simulink model "Task2_2"  (R2021a)
settings: Solver=VariableStepAuto  StartTime=0.0  StopTime=stop_time  RelTol=1e-3
values from neighbouring files (symbols this model uses):
  i_sd_ref = i_sd_mat(end)    [Code2021_Jo_Saleh.m]    (also in ExeRet21.m.m)
  i_sq_ref = i_sq_mat(end)    [Code2021_Jo_Saleh.m]    (also in ExeRet21.m.m)
  Kd_i = Rs * Kd_p / Lsd    (= -20)    [Code2021_Jo_Saleh.m]    (also in ExeRet21.m.m)
  Kd_p = - Lsd / tau_i    (= -2)    [Code2021_Jo_Saleh.m]    (also in ExeRet21.m.m)
  Kq_i = Rs * Kq_p / Lsq    (= -20)    [Code2021_Jo_Saleh.m]    (also in ExeRet21.m.m)
  Kq_p = - Lsq / tau_i    (= -2.66666666667)    [Code2021_Jo_Saleh.m]    (also in ExeRet21.m.m)
  Lsd = 6e-3    (= 0.006)    [Code2021_Jo_Saleh.m]    (also in ExeRet21.m.m)
  Lsq = 8e-3    (= 0.008)    [Code2021_Jo_Saleh.m]    (also in ExeRet21.m.m)
  Phi_m = 17.3    [Code2021_Jo_Saleh.m]    (also in ExeRet21.m.m)
  Ptur = 3.5e6    (= 3500000)    [Code2021_Jo_Saleh.m]    (also in ExeRet21.m.m)
  Rs = 60e-3    (= 0.06)    [Code2021_Jo_Saleh.m]    (also in ExeRet21.m.m)
  Vdc = 6e3    (= 6000)    [Code2021_Jo_Saleh.m]    (also in ExeRet21.m.m)
  we = wm * (p / 2)    (= 188.495559215)    [Code2021_Jo_Saleh.m]    (also in ExeRet21.m.m)
libraries: pid_lib x2
settings Model: Creator=Tomo  LastModifiedBy=Tomo
settings SolverCC: AlgebraicLoopSolver=TrustRegion
settings DebuggingCC: SFMachineParentedDataDiag=warning

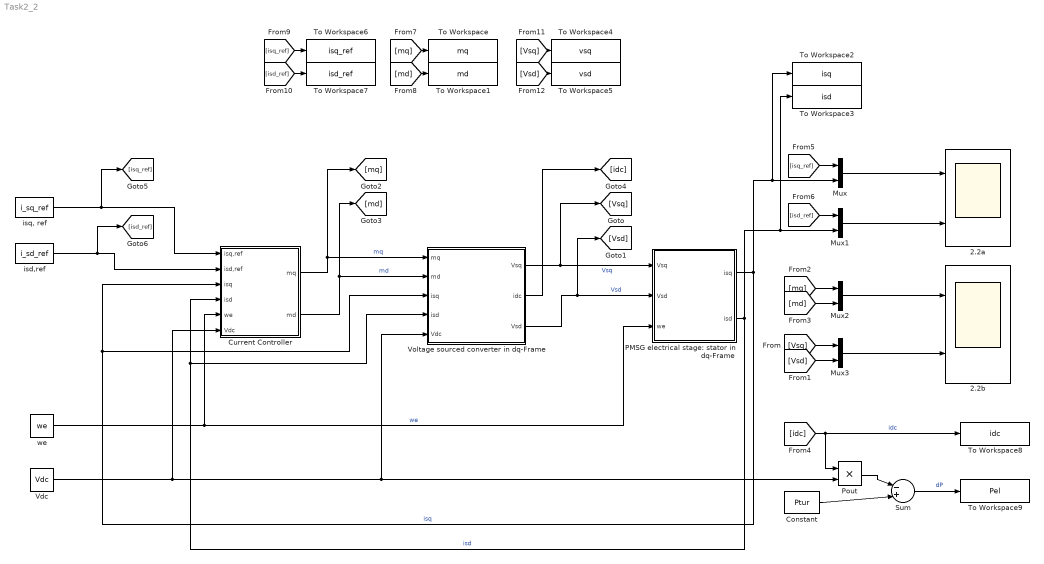
== system Task2_2 ==
  2.2a : Scope  NumInputPorts=2
  2.2b : Scope  NumInputPorts=2
  Constant : Constant  Value=Ptur
  Current Controller : Subsystem
  Mux{,1..3} (4 alike) : Mux  Inputs=2
  PMSG electrical stage: stator in dq-Frame : Subsystem
  Pout : Product
  Sum : Sum  Inputs=|-+|
  To Workspace : ToWorkspace  VariableName=mq  SampleTime=-1
  To Workspace1 : ToWorkspace  VariableName=md  SampleTime=-1
  To Workspace2 : ToWorkspace  VariableName=isq  SampleTime=-1
  To Workspace3 : ToWorkspace  VariableName=isd  SampleTime=-1
  To Workspace4 : ToWorkspace  VariableName=vsq  SampleTime=-1
  To Workspace5 : ToWorkspace  VariableName=vsd  SampleTime=-1
  To Workspace6 : ToWorkspace  VariableName=isq_ref  SampleTime=-1
  To Workspace7 : ToWorkspace  VariableName=isd_ref  SampleTime=-1
  To Workspace8 : ToWorkspace  VariableName=idc  SampleTime=-1
  To Workspace9 : ToWorkspace  VariableName=Pel  SampleTime=-1
  Vdc : Constant  Value=Vdc
  Voltage sourced converter in dq-Frame : Subsystem
  isd,ref : Constant  Value=i_sd_ref
  "isq, ref" : Constant  Value=i_sq_ref
  we : Constant  Value=we
  wires:
  "isq, ref"/1 -> [isq_ref], Current Controller/1(isq,ref)
  isd,ref/1 -> [isd_ref], Current Controller/2(isd,ref)
  PMSG electrical stage: stator in dq-Frame/1(isq) -> To Workspace2/1, Mux/2, Voltage sourced converter in dq-Frame/3(isq), Current Controller/3(isq)  "isq"
  PMSG electrical stage: stator in dq-Frame/2(isd) -> To Workspace3/1, Mux1/2, Voltage sourced converter in dq-Frame/4(isd), Current Controller/4(isd)  "isd"
  we/1 -> PMSG electrical stage: stator in dq-Frame/3(we), Current Controller/5(we)  "we"
  Vdc/1 -> Voltage sourced converter in dq-Frame/5(Vdc), Pout/2, Current Controller/6(Vdc)
  Current Controller/1(mq) -> [mq], Voltage sourced converter in dq-Frame/1(mq)  "mq"
  Current Controller/2(md) -> [md], Voltage sourced converter in dq-Frame/2(md)  "md"
  Voltage sourced converter in dq-Frame/1(Vsq) -> PMSG electrical stage: stator in dq-Frame/1(Vsq), [Vsq]  "Vsq"
  Voltage sourced converter in dq-Frame/3(Vsd) -> [Vsd], PMSG electrical stage: stator in dq-Frame/2(Vsd)  "Vsd"
  [Vsq] -> Mux3/1
  Voltage sourced converter in dq-Frame/2(idc) -> [idc]
  [idc] -> To Workspace8/1, Pout/1  "idc"
  [isq_ref] -> Mux/1
  Mux/1 -> 2.2a/1
  Mux1/1 -> 2.2a/2
  [isd_ref] -> Mux1/1
  Mux2/1 -> 2.2b/1
  Mux3/1 -> 2.2b/2
  [Vsd] -> Mux3/2
  [md] -> Mux2/2
  [mq] -> Mux2/1
  Constant/1 -> Sum/2
  Pout/1 -> Sum/1
  Sum/1 -> To Workspace9/1  "dP"
  [mq] -> To Workspace/1
  [md] -> To Workspace1/1
  [Vsd] -> To Workspace5/1
  [Vsq] -> To Workspace4/1
  [isq_ref] -> To Workspace6/1
  [isd_ref] -> To Workspace7/1

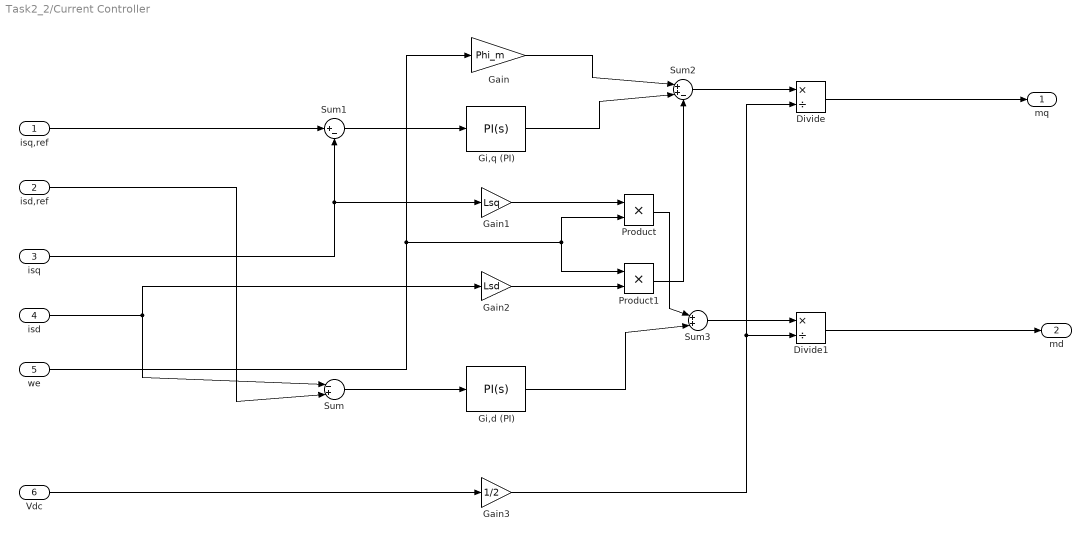
== system Task2_2/Current Controller ==
  isq,ref : Inport
  isd,ref : Inport  Port=2
  isq : Inport  Port=3
  isd : Inport  Port=4
  we : Inport  Port=5
  Vdc : Inport  Port=6
  Divide : Product  Inputs=*/
  Divide1 : Product  Inputs=*/
  Gain : Gain  Gain=Phi_m
  Gain1 : Gain  Gain=Lsq
  Gain2 : Gain  Gain=Lsd
  Gain3 : Gain  Gain=1/2
  Gi,d (PI) : pid_lib/PID Controller  Controller=PI  Form=Parallel  TimeDomain=Continuous-time  UseExternalTs=off  SampleTime=-1  IntegratorMethod=Forward Euler  FilterMethod=Forward Euler  ControllerParametersSource=internal  P=Kd_p  I=Kd_i  D=0  UseFilter=on  N=100  TunerSelectOption=Transfer Function Based (PID Tuner App)  InitialConditionSource=internal  InitialConditionForIntegrator=0  InitialConditionForFilter=0  DifferentiatorICPrevScaledInput=0  ExternalReset=none  TrackingMode=off  Kt=1  LimitOutput=off  SatLimitsSource=internal  UpperSaturationLimit=inf  LowerSaturationLimit=-inf  LinearizeAsGain=on  AntiWindupMode=none  Kb=1  POutMin=[]  POutMax=[]  IOutMin=[]  IOutMax=[]  DOutMin=[]  DOutMax=[]  NOutMin=[]  NOutMax=[]  SumOutMin=[]  SumOutMax=[]  SaturationOutMin=[]  SaturationOutMax=[]  PParamMin=[]  PParamMax=[]  IParamMin=[]  IParamMax=[]  DParamMin=[]  DParamMax=[]  NParamMin=[]  NParamMax=[]  KbParamMin=[]  KbParamMax=[]  KtParamMin=[]  KtParamMax=[]  KbOutMin=[]  KbOutMax=[]  KtOutMin=[]  KtOutMax=[]  IntegratorOutMin=[]  IntegratorOutMax=[]  FilterOutMin=[]  FilterOutMax=[]  SumI1OutMin=[]  SumI1OutMax=[]  SumI2OutMin=[]  SumI2OutMax=[]  SumI3OutMin=[]  SumI3OutMax=[]  SumI4OutMin=[]  SumI4OutMax=[]  SumDOutMin=[]  SumDOutMax=[]  DifferentiatorOutMin=[]  DifferentiatorOutMax=[]  FilterDiffOutCoefMin=[]  FilterDiffOutCoefMax=[]  ReciprocalOutMin=[]  ReciprocalOutMax=[]  SumDenOutMin=[]  SumDenOutMax=[]  SumNumOutMin=[]  SumNumOutMax=[]  DivideOutMin=[]  DivideOutMax=[]  UdiffTsProdOutMin=[]  UdiffTsProdOutMax=[]  NTsProdOutMin=[]  NTsProdOutMax=[]  UintegralTsProdOutMin=[]  UintegralTsProdOutMax=[]  UngainTsProdOutMin=[]  UngainTsProdOutMax=[]  IntegratorContinuousStateAttributes=''  IntegratorStateMustResolveToSignalObject=off  IntegratorRTWStateStorageClass=Auto  FilterContinuousStateAttributes=''  FilterStateMustResolveToSignalObject=off  FilterRTWStateStorageClass=Auto  ParallelPVariant=InternalParameters  IdealPVariant=Disabled  IVariant=InternalParameters  DVariant=Disabled  IntegratorVariant=Continuous  SatVariant=Disabled  AWVariant=Passthrough  PCopyVariant=Disabled  TRVariant=Disabled  FdbkBlocksVariant=Forward  IdealPFdbkVariant=Disabled  SatFdbkVariant=Disabled  DerivativeFilterVariant=Disabled  NVariant=Disabled  NCopyVariant=Disabled_SignalSpec  FilterICVariant=Disabled  IntegratorICVariant=InternalICs  ExternalResetVariant=Disabled  TRSumVariant=Passthrough  SumFdbkVariant=Disabled  SumVariant=Sum_PI  TsampFilterVariant=InternalTs  TsampNgainVariant=Passthrough  TsampIntegralVariant=Passthrough  ExternalSaturationOutDataTypeStr=Inherit: Same as second input
  Gi,q (PI) : pid_lib/PID Controller  Controller=PI  Form=Parallel  TimeDomain=Continuous-time  UseExternalTs=off  SampleTime=-1  IntegratorMethod=Forward Euler  FilterMethod=Forward Euler  ControllerParametersSource=internal  P=Kq_p  I=Kq_i  D=0  UseFilter=on  N=100  TunerSelectOption=Transfer Function Based (PID Tuner App)  InitialConditionSource=internal  InitialConditionForIntegrator=0  InitialConditionForFilter=0  DifferentiatorICPrevScaledInput=0  ExternalReset=none  TrackingMode=off  Kt=1  LimitOutput=off  SatLimitsSource=internal  UpperSaturationLimit=inf  LowerSaturationLimit=-inf  LinearizeAsGain=on  AntiWindupMode=none  Kb=1  POutMin=[]  POutMax=[]  IOutMin=[]  IOutMax=[]  DOutMin=[]  DOutMax=[]  NOutMin=[]  NOutMax=[]  SumOutMin=[]  SumOutMax=[]  SaturationOutMin=[]  SaturationOutMax=[]  PParamMin=[]  PParamMax=[]  IParamMin=[]  IParamMax=[]  DParamMin=[]  DParamMax=[]  NParamMin=[]  NParamMax=[]  KbParamMin=[]  KbParamMax=[]  KtParamMin=[]  KtParamMax=[]  KbOutMin=[]  KbOutMax=[]  KtOutMin=[]  KtOutMax=[]  IntegratorOutMin=[]  IntegratorOutMax=[]  FilterOutMin=[]  FilterOutMax=[]  SumI1OutMin=[]  SumI1OutMax=[]  SumI2OutMin=[]  SumI2OutMax=[]  SumI3OutMin=[]  SumI3OutMax=[]  SumI4OutMin=[]  SumI4OutMax=[]  SumDOutMin=[]  SumDOutMax=[]  DifferentiatorOutMin=[]  DifferentiatorOutMax=[]  FilterDiffOutCoefMin=[]  FilterDiffOutCoefMax=[]  ReciprocalOutMin=[]  ReciprocalOutMax=[]  SumDenOutMin=[]  SumDenOutMax=[]  SumNumOutMin=[]  SumNumOutMax=[]  DivideOutMin=[]  DivideOutMax=[]  UdiffTsProdOutMin=[]  UdiffTsProdOutMax=[]  NTsProdOutMin=[]  NTsProdOutMax=[]  UintegralTsProdOutMin=[]  UintegralTsProdOutMax=[]  UngainTsProdOutMin=[]  UngainTsProdOutMax=[]  IntegratorContinuousStateAttributes=''  IntegratorStateMustResolveToSignalObject=off  IntegratorRTWStateStorageClass=Auto  FilterContinuousStateAttributes=''  FilterStateMustResolveToSignalObject=off  FilterRTWStateStorageClass=Auto  ParallelPVariant=InternalParameters  IdealPVariant=Disabled  IVariant=InternalParameters  DVariant=Disabled  IntegratorVariant=Continuous  SatVariant=Disabled  AWVariant=Passthrough  PCopyVariant=Disabled  TRVariant=Disabled  FdbkBlocksVariant=Forward  IdealPFdbkVariant=Disabled  SatFdbkVariant=Disabled  DerivativeFilterVariant=Disabled  NVariant=Disabled  NCopyVariant=Disabled_SignalSpec  FilterICVariant=Disabled  IntegratorICVariant=InternalICs  ExternalResetVariant=Disabled  TRSumVariant=Passthrough  SumFdbkVariant=Disabled  SumVariant=Sum_PI  TsampFilterVariant=InternalTs  TsampNgainVariant=Passthrough  TsampIntegralVariant=Passthrough  ExternalSaturationOutDataTypeStr=Inherit: Same as second input
  Product : Product
  Product1 : Product
  Sum : Sum  Inputs=|-+|
  Sum1 : Sum  Inputs=|+-
  Sum2 : Sum  Inputs=|++-
  Sum3 : Sum  Inputs=|++|
  mq : Outport
  md : Outport  Port=2
  wires:
  Gain3/1 -> Divide/2, Divide1/2
  we/1 -> Gain/1, Product1/1, Product/2
  Sum/1 -> Gi,d (PI)/1
  Vdc/1 -> Gain3/1
  Sum3/1 -> Divide1/1
  isq/1 -> Gain1/1, Sum1/2
  Sum1/1 -> Gi,q (PI)/1
  Gain/1 -> Sum2/1
  Gain2/1 -> Product1/2
  isd,ref/1 -> Sum/2
  Sum2/1 -> Divide/1
  Gi,d (PI)/1 -> Sum3/2
  Product/1 -> Sum3/1
  Product1/1 -> Sum2/3
  Gain1/1 -> Product/1
  isq,ref/1 -> Sum1/1
  Gi,q (PI)/1 -> Sum2/2
  Divide/1 -> mq/1
  isd/1 -> Gain2/1, Sum/1
  Divide1/1 -> md/1

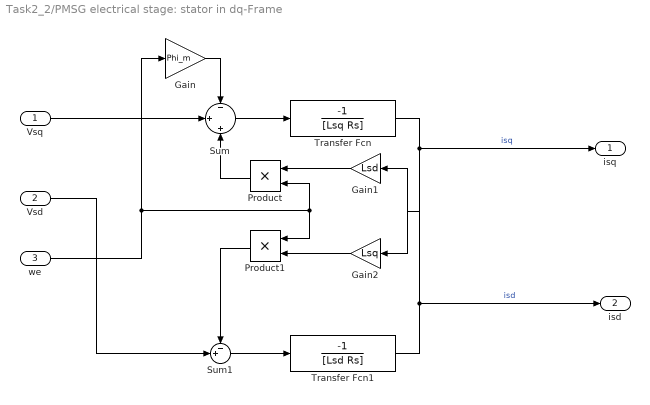
== system Task2_2/PMSG electrical stage: stator in dq-Frame ==
  Vsq : Inport
  Vsd : Inport  Port=2
  we : Inport  Port=3
  Gain : Gain  Gain=Phi_m
  Gain1 : Gain  Gain=Lsd
  Gain2 : Gain  Gain=Lsq
  Product : Product
  Product1 : Product
  Sum : Sum  Inputs=-|+|+
  Sum1 : Sum  Inputs=-+|
  Transfer Fcn : TransferFcn  Numerator=[-1]  Denominator=[Lsq Rs]
  Transfer Fcn1 : TransferFcn  Numerator=[-1]  Denominator=[Lsd Rs]
  isq : Outport
  isd : Outport  Port=2
  wires:
  Sum/1 -> Transfer Fcn/1
  Product/1 -> Sum/3
  Gain/1 -> Sum/1
  we/1 -> Gain/1, Product/2, Product1/1
  Transfer Fcn1/1 -> Gain1/1, isd/1  "isd"
  Vsq/1 -> Sum/2
  Transfer Fcn/1 -> Gain2/1, isq/1  "isq"
  Product1/1 -> Sum1/1
  Sum1/1 -> Transfer Fcn1/1
  Vsd/1 -> Sum1/2
  Gain1/1 -> Product/1
  Gain2/1 -> Product1/2

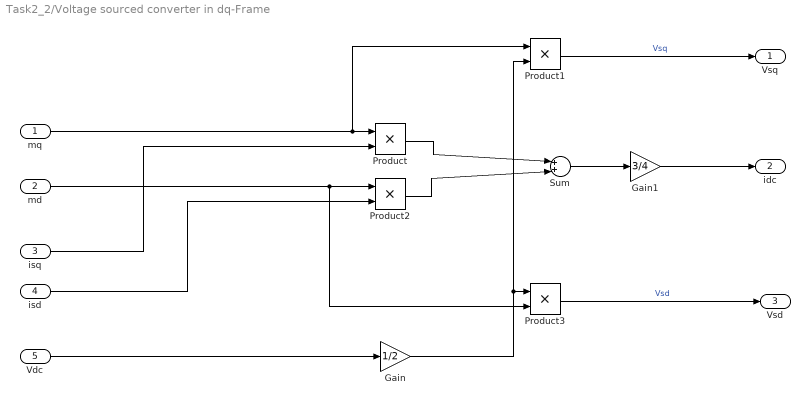
== system Task2_2/Voltage sourced converter in dq-Frame ==
  mq : Inport
  md : Inport  Port=2
  isq : Inport  Port=3
  isd : Inport  Port=4
  Vdc : Inport  Port=5
  Gain : Gain  Gain=1/2
  Gain1 : Gain  Gain=3/4
  Product{,1..3} (4 alike) : Product
  Sum : Sum  Inputs=|++|
  Vsq : Outport
  idc : Outport  Port=2
  Vsd : Outport  Port=3
  wires:
  Product2/1 -> Sum/2
  mq/1 -> Product1/1, Product/1
  Gain/1 -> Product1/2, Product3/1
  isd/1 -> Product2/2
  Vdc/1 -> Gain/1
  md/1 -> Product3/2, Product2/1
  Product3/1 -> Vsd/1  "Vsd"
  Product1/1 -> Vsq/1  "Vsq"
  Sum/1 -> Gain1/1
  isq/1 -> Product/2
  Product/1 -> Sum/1
  Gain1/1 -> idc/1
